simulink model "RobotStepID"  (R2022b)
settings: Solver=VariableStepAuto  StartTime=0.0  StopTime=10.0  RelTol=1e-3
undefined symbols (not defined in the file): kPhi, kV, om_nPhi, om_nV, setaPhi, setaV
settings Model: Creator=Charles A Vath  LastModifiedBy=Charles A Vath

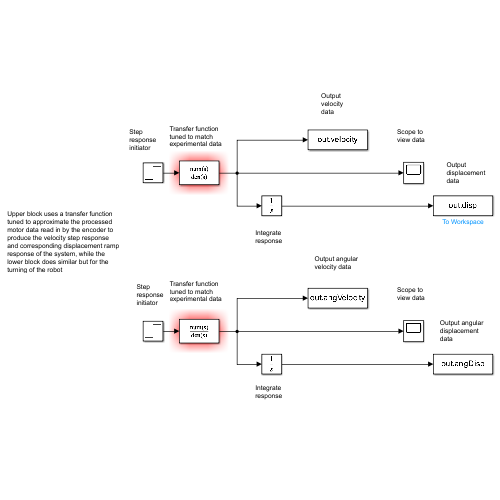
[thumbnail: Simulink's stored preview of the top-level diagram]
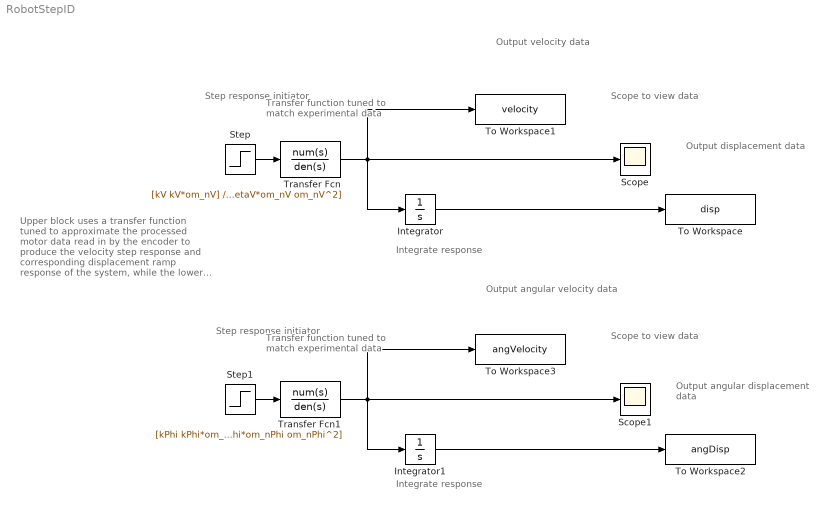
== system RobotStepID ==
  note: Upper block uses a transfer function tuned to approximate the processed motor data read in by the encoder to produce the velocity step response and corresponding displacement ramp response of the system, while the lower block does similar but for the turning of the robot
  note: Step response initiator
  note: Output velocity data
  note: Integrate response
  note: Integrate response
  note: Scope to view data
  note: Output displacement data
  note: Step response initiator
  note: Transfer function tuned to match experimental data
  note: Transfer function tuned to match experimental data
  note: Output angular velocity data
  note: Scope to view data
  note: Output angular displacement data
  Integrator : Integrator
  Integrator1 : Integrator
  Scope : Scope
  Scope1 : Scope
  Step : Step  SampleTime=0
  Step1 : Step  SampleTime=0
  To Workspace : ToWorkspace  VariableName=disp  SaveFormat=Timeseries  SampleTime=-1
  To Workspace1 : ToWorkspace  VariableName=velocity  SaveFormat=Timeseries  SampleTime=-1
  To Workspace2 : ToWorkspace  VariableName=angDisp  SaveFormat=Timeseries  SampleTime=-1
  To Workspace3 : ToWorkspace  VariableName=angVelocity  SaveFormat=Timeseries  SampleTime=-1
  Transfer Fcn : TransferFcn  Numerator=[kV kV*om_nV]  Denominator=[1 2*setaV*om_nV om_nV^2]
  Transfer Fcn1 : TransferFcn  Numerator=[kPhi kPhi*om_nPhi]  Denominator=[1 2*setaPhi*om_nPhi om_nPhi^2]
  wires:
  Integrator/1 -> To Workspace/1
  Transfer Fcn/1 -> Integrator/1, To Workspace1/1, Scope/1
  Step/1 -> Transfer Fcn/1
  Integrator1/1 -> To Workspace2/1
  Transfer Fcn1/1 -> Integrator1/1, To Workspace3/1, Scope1/1
  Step1/1 -> Transfer Fcn1/1
